simulink model "TimeTrajLinear"  (R2025b)
settings: Solver=ode4  StartTime=0.0  StopTime=110  FixedStep=0.1  RelTol=1e-3
settings Model: Creator=20241588  LastModifiedBy=20241588

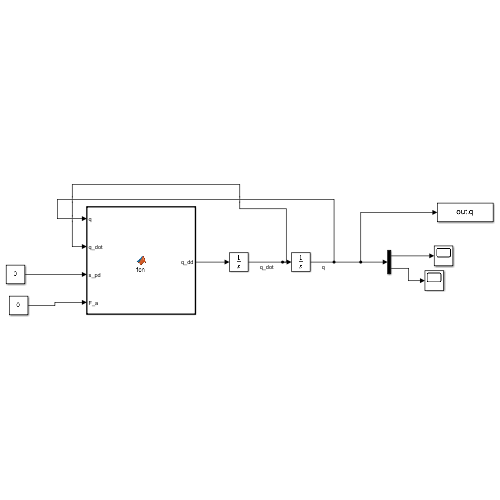
[thumbnail: Simulink's stored preview of the top-level diagram]
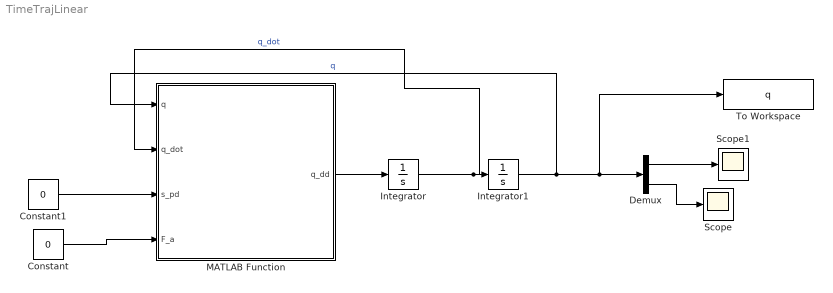
== system TimeTrajLinear ==
  Constant : Constant  Value=0
  Constant1 : Constant  Value=0
  Demux : Demux  Outputs=2
  Integrator : Integrator  InitialCondition=[0,0]
  Integrator1 : Integrator  InitialCondition=[11.5,pi/3]
  MATLAB Function : MATLAB Function  TreatAsAtomicUnit=on
  Scope : Scope
      settings: ActiveDisplayYMinimum=0.22511347109079183  ActiveDisplayYMaximum=2.3883257204682788
  Scope1 : Scope
      settings: ActiveDisplayYMinimum=11.440410710528061  ActiveDisplayYMaximum=13.030120965311056
  To Workspace : ToWorkspace  VariableName=q  SampleTime=-1
  wires:
  MATLAB Function/1(q_dd) -> Integrator/1
  Integrator/1 -> MATLAB Function/2(q_dot), Integrator1/1  "q_dot"
  Integrator1/1 -> To Workspace/1, Demux/1, MATLAB Function/1(q)  "q"
  Constant/1 -> MATLAB Function/4(F_a)
  Constant1/1 -> MATLAB Function/3(s_pd)
  Demux/2 -> Scope/1
  Demux/1 -> Scope1/1

== matlab function TimeTrajLinear/MATLAB Function ==
  data: q input; q_dd output double size=2; q_dot input; s_pd input; F_a input
function q_dd = fcn(q, q_dot, s_pd, F_a)
% q_dd = fcn(q, q_dot, s_pd, F_a)
% q      = [x; theta]
% q_dot  = [x_dot; theta_dot]
% s_pd   = (unused here, but kept for interface compatibility)
% F_a    = actuator force input

    % constants
    g = 9.81;
    L0 = 30;
    L1 = 25;
    L2 = 10;
    m0 = 10^4;
    m1 = 10^4;
    m2 = 2000;
    m3 = 500;
    dx = 200;
    dw = 2000;
    dphi = 2;
    k_theta = 200;
    theta_ref = 0;
    d_theta = 10;
    kx = 7000;
    Lx = 12.5;

    % equilibrium angle (the big fraction)
    phi0 = 7045509688949645/4503599627370496;

    % generalised coordinates
    x     = q(1);
    theta = q(2);

    x_dot     = q_dot(1);
    theta_dot = q_dot(2);

    % In your setup phi is treated as constant
    phi     = 0;
    phi_dot = 0;

    % input force
    Fa = F_a;

    % ---- Mass matrix M (2x2) ----
    s = sin(phi - phi0);  % since phi = 0, this is sin(-phi0), a constant

    M = [ ...
        2500,        -5000 * s; ...
       -5000 * s,     50000     ...
    ];

    % ---- Forcing vector F (2x1) ----
    F = zeros(2,1);

    % First equation
    F(1) = Fa ...
           - 7000 * x ...
           - 200  * x_dot ...
           + 2000 * theta_dot * sin(phi - phi0) ...
           + 87500;

    % Second equation
    F(2) = 10 * phi_dot ...
           - 20010 * theta_dot ...
           - (theta - phi0) * (49050 * sin(phi0) + 200);

    % Solve M * q_dd = F  → q_dd = M\F
    q_dd = M \ F;

end
